simulink model "DPID_EKF"  (R2017a)
settings: Solver=ode1  StartTime=0.0  StopTime=125  FixedStep=block_sample_time  RelTol=1e-3
values from neighbouring files (symbols this model uses):
  GAMAin = 100    [model_params.m]
  Ks = 0.012    [model_params.m]
  MUmax = 0.55    [model_params.m]
  T0 = 0.0056    [dlqr_reg.m]    (also in model_params.m)
  Ysx = 0.5    [model_params.m]
undefined symbols (not defined in the file or in its folder): serial
libraries: instrumentlib x3
settings Model: Creator=user  LastModifiedBy=user

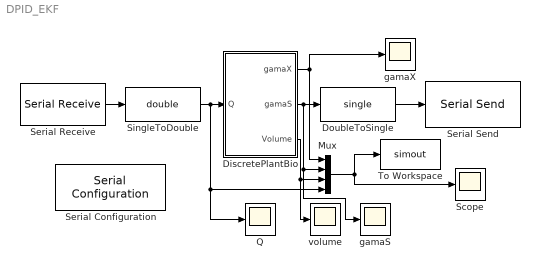
== system DPID_EKF ==
  DiscretePlantBio : Subsystem
  DoubleToSingle : DataTypeConversion  OutDataTypeStr=single
  Mux : Mux
  Q : Scope
  Scope : Scope
  Serial Configuration : instrumentlib/Serial Configuration  Priority=-200000  ComPortMenu=<Please select a port...>  ComPort=COM3  ObjConstructor=serial('COM3');  BaudRate=9600  DataBits=8  Parity=none  StopBits=1  FlowControl=none  Timeout=10  ByteOrder=LittleEndian
  Serial Receive : instrumentlib/Serial Receive  ComPortMenu=<Please select a port...>  ComPort=COM3  ObjConstructor=serial('COM3');  Terminator=<none>  DataSize=1  DataType=single  EnableBlockingMode=on  ActionDataUnavailable=Output last received value  CustomValue=0  SampleTime=0.1
  Serial Send : instrumentlib/Serial Send  ComPortMenu=<Please select a port...>  ComPort=COM3  ObjConstructor=serial('COM3');  Terminator=<none>  EnableBlockingMode=on
  SingleToDouble : DataTypeConversion  OutDataTypeStr=double
  To Workspace : ToWorkspace  VariableName=simout  SampleTime=-1
  "gamaS " : Scope
  gamaX : Scope
  "volume " : Scope
  wires:
  Serial Receive/1 -> SingleToDouble/1
  SingleToDouble/1 -> Q/1, Mux/4, DiscretePlantBio/1(Q)
  Mux/1 -> Scope/1, To Workspace/1
  DiscretePlantBio/2(gamaS) -> DoubleToSingle/1, Mux/2, "gamaS "/1
  DoubleToSingle/1 -> Serial Send/1
  DiscretePlantBio/3(Volume) -> "volume "/1, Mux/3
  DiscretePlantBio/1(gamaX) -> Mux/1, gamaX/1

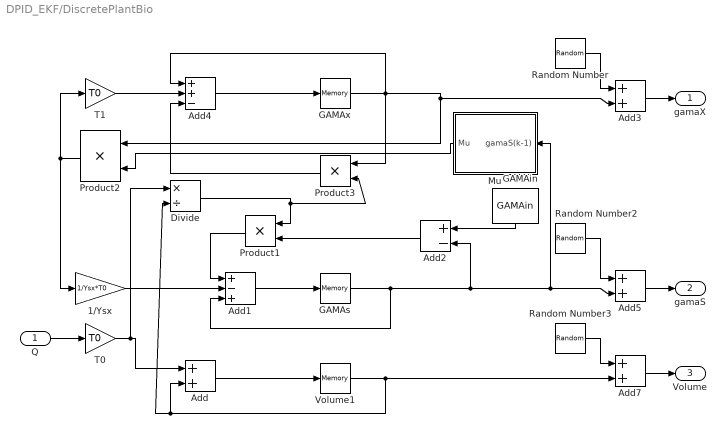
== system DPID_EKF/DiscretePlantBio ==
  Q : Inport
  1/Ysx : Gain  Gain=1/Ysx*T0
  Add{,3,5,7} (4 alike) : Sum
  Add1 : Sum  Inputs=+-+
  Add2 : Sum  Inputs=+-
  Add4 : Sum  Inputs=++-
  Divide : Product  Inputs=*/
  GAMAin : Constant  Value=GAMAin
  GAMAs : Memory  X0=0.81
  GAMAx : Memory  X0=1.25
  Mu : Subsystem
  Product1 : Product  RndMeth=Zero
  Product2 : Product  RndMeth=Zero
  Product3 : Product  RndMeth=Zero
  Random Number : RandomNumber  Variance=0.0025  Seed=34645  SampleTime=0.1
  Random Number2 : RandomNumber  Variance=0.001  Seed=454645  SampleTime=0.1
  Random Number3 : RandomNumber  Variance=0.001  Seed=4546  SampleTime=0.1
  T0 : Gain  Gain=T0
  T1 : Gain  Gain=T0
  Volume1 : Memory  X0=1.35
  gamaX : Outport
  gamaS : Outport  Port=2
  Volume : Outport  Port=3
  wires:
  Product1/1 -> Add1/1
  Add2/1 -> Product1/2
  GAMAin/1 -> Add2/1
  1/Ysx/1 -> Add1/2
  Product2/1 -> 1/Ysx/1, T1/1
  Product3/1 -> Add4/3
  Add1/1 -> GAMAs/1
  Add4/1 -> GAMAx/1
  Mu/1(Mu) -> Product2/2
  GAMAs/1 -> Add2/2, Mu/1(gamaS(k-1)), Add5/2, Add1/3
  GAMAx/1 -> Product3/1, Add4/1, Product2/1, Add3/2
  Add/1 -> Volume1/1
  Volume1/1 -> Divide/2, Add/2, Add7/2
  T0/1 -> Add/1, Divide/1
  Divide/1 -> Product1/1, Product3/2
  T1/1 -> Add4/2
  Add3/1 -> gamaX/1
  Add5/1 -> gamaS/1
  Q/1 -> T0/1
  Add7/1 -> Volume/1
  Random Number2/1 -> Add5/1
  Random Number/1 -> Add3/1
  Random Number3/1 -> Add7/1

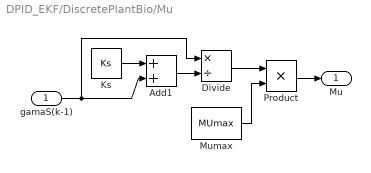
== system DPID_EKF/DiscretePlantBio/Mu ==
  gamaS(k-1) : Inport
  Add1 : Sum
  Divide : Product  Inputs=*/
  Ks : Constant  Value=Ks
  Mumax : Constant  Value=MUmax
  Product : Product  RndMeth=Zero
  Mu : Outport
  wires:
  Ks/1 -> Add1/1
  Add1/1 -> Divide/2
  Divide/1 -> Product/1
  Mumax/1 -> Product/2
  Product/1 -> Mu/1
  gamaS(k-1)/1 -> Add1/2, Divide/1
